simulink model "Wanderwellen_Leitungsmodell"  (R2022a)
settings: Solver=VariableStepAuto  StartTime=0.0  StopTime=0.05  RelTol=1e-3
model workspace (MAT data in the model file):
  C_impedanz = 1
  C_quelle = 1
  Delta_C = 2e-09
  Delta_G = 5000000
  Delta_L = 0.000228
  Delta_R = 0.048
  L_impedanz = 1
  L_quelle = 1
  R_impedanz = 0
  R_quelle = 0
  U = 20000
  U_type = 1
  Z_abschluss_type = 1
  Z_quelle_type = 1
  f = 50
  laenge = 0.2
  n_seg = 1
libraries: fl_lib x617, nesl_utility x207, ee_lib x3
(part 4 of 6)

== system Wanderwellen_Leitungsmodell/10 Leitungs-ESBs Nr. 3/Leitungs-ESB 6 ==
  Capacitor : fl_lib/Electrical/Electrical Elements/Capacitor  c=Delta_C F  r=1e-6 Ohm  g=0 1/Ohm  i_specify=off  i_priority=None  i=0 A  i_nominal_specify=off  i_nominal_unit=A  i_nominal_value=1  v_specify=off  v_priority=None  v=0 V  v_nominal_specify=off  v_nominal_unit=V  v_nominal_value=1  vc_specify=off  vc_priority=High  vc=0 V  vc_nominal_specify=off  vc_nominal_unit=V  vc_nominal_value=1
      settings: SourceProductBaseCode=PW,SS,VE
  Inductor : fl_lib/Electrical/Electrical Elements/Inductor  l=Delta_L H  r=0 Ohm  g=1e-9 1/Ohm  i_specify=off  i_priority=None  i=0 A  i_nominal_specify=off  i_nominal_unit=A  i_nominal_value=1  v_specify=off  v_priority=None  v=0 V  v_nominal_specify=off  v_nominal_unit=V  v_nominal_value=1  i_L_specify=off  i_L_priority=High  i_L=0 A  i_L_nominal_specify=off  i_L_nominal_unit=A  i_L_nominal_value=1
      settings: SourceProductBaseCode=PW,SS,VE
  Resistor : fl_lib/Electrical/Electrical Elements/Resistor  R=Delta_R Ohm  i_specify=off  i_priority=None  i=0 A  i_nominal_specify=off  i_nominal_unit=A  i_nominal_value=1  v_specify=off  v_priority=None  v=0 V  v_nominal_specify=off  v_nominal_unit=V  v_nominal_value=1
      settings: SourceProductBaseCode=PW,SS,VE
  Resistor1 : fl_lib/Electrical/Electrical Elements/Resistor  R=Delta_G Ohm  i_specify=off  i_priority=None  i=0 A  i_nominal_specify=off  i_nominal_unit=A  i_nominal_value=1  v_specify=off  v_priority=None  v=0 V  v_nominal_specify=off  v_nominal_unit=V  v_nominal_value=1
      settings: SourceProductBaseCode=PW,SS,VE
  L_in : PMIOPort  Side=Left
  N_in : PMIOPort  Port=2  Side=Left
  L_out : PMIOPort  Port=3  Side=Right
  N_out : PMIOPort  Port=4  Side=Right
  connections:
  Capacitor/LConn1 -- Resistor1/LConn1 -- Inductor/RConn1 -- L_out/RConn1
  Inductor/LConn1 -- Resistor/RConn1
  L_in/RConn1 -- Resistor/LConn1
  Resistor1/RConn1 -- N_in/RConn1 -- N_out/RConn1 -- Capacitor/RConn1

== system Wanderwellen_Leitungsmodell/10 Leitungs-ESBs Nr. 3/Leitungs-ESB 7 ==
  Capacitor : fl_lib/Electrical/Electrical Elements/Capacitor  c=Delta_C F  r=1e-6 Ohm  g=0 1/Ohm  i_specify=off  i_priority=None  i=0 A  i_nominal_specify=off  i_nominal_unit=A  i_nominal_value=1  v_specify=off  v_priority=None  v=0 V  v_nominal_specify=off  v_nominal_unit=V  v_nominal_value=1  vc_specify=off  vc_priority=High  vc=0 V  vc_nominal_specify=off  vc_nominal_unit=V  vc_nominal_value=1
      settings: SourceProductBaseCode=PW,SS,VE
  Inductor : fl_lib/Electrical/Electrical Elements/Inductor  l=Delta_L H  r=0 Ohm  g=1e-9 1/Ohm  i_specify=off  i_priority=None  i=0 A  i_nominal_specify=off  i_nominal_unit=A  i_nominal_value=1  v_specify=off  v_priority=None  v=0 V  v_nominal_specify=off  v_nominal_unit=V  v_nominal_value=1  i_L_specify=off  i_L_priority=High  i_L=0 A  i_L_nominal_specify=off  i_L_nominal_unit=A  i_L_nominal_value=1
      settings: SourceProductBaseCode=PW,SS,VE
  Resistor : fl_lib/Electrical/Electrical Elements/Resistor  R=Delta_R Ohm  i_specify=off  i_priority=None  i=0 A  i_nominal_specify=off  i_nominal_unit=A  i_nominal_value=1  v_specify=off  v_priority=None  v=0 V  v_nominal_specify=off  v_nominal_unit=V  v_nominal_value=1
      settings: SourceProductBaseCode=PW,SS,VE
  Resistor1 : fl_lib/Electrical/Electrical Elements/Resistor  R=Delta_G Ohm  i_specify=off  i_priority=None  i=0 A  i_nominal_specify=off  i_nominal_unit=A  i_nominal_value=1  v_specify=off  v_priority=None  v=0 V  v_nominal_specify=off  v_nominal_unit=V  v_nominal_value=1
      settings: SourceProductBaseCode=PW,SS,VE
  L_in : PMIOPort  Side=Left
  N_in : PMIOPort  Port=2  Side=Left
  L_out : PMIOPort  Port=3  Side=Right
  N_out : PMIOPort  Port=4  Side=Right
  connections:
  Capacitor/LConn1 -- Resistor1/LConn1 -- Inductor/RConn1 -- L_out/RConn1
  Inductor/LConn1 -- Resistor/RConn1
  L_in/RConn1 -- Resistor/LConn1
  Resistor1/RConn1 -- N_in/RConn1 -- N_out/RConn1 -- Capacitor/RConn1

== system Wanderwellen_Leitungsmodell/10 Leitungs-ESBs Nr. 3/Leitungs-ESB 8 ==
  Capacitor : fl_lib/Electrical/Electrical Elements/Capacitor  c=Delta_C F  r=1e-6 Ohm  g=0 1/Ohm  i_specify=off  i_priority=None  i=0 A  i_nominal_specify=off  i_nominal_unit=A  i_nominal_value=1  v_specify=off  v_priority=None  v=0 V  v_nominal_specify=off  v_nominal_unit=V  v_nominal_value=1  vc_specify=off  vc_priority=High  vc=0 V  vc_nominal_specify=off  vc_nominal_unit=V  vc_nominal_value=1
      settings: SourceProductBaseCode=PW,SS,VE
  Inductor : fl_lib/Electrical/Electrical Elements/Inductor  l=Delta_L H  r=0 Ohm  g=1e-9 1/Ohm  i_specify=off  i_priority=None  i=0 A  i_nominal_specify=off  i_nominal_unit=A  i_nominal_value=1  v_specify=off  v_priority=None  v=0 V  v_nominal_specify=off  v_nominal_unit=V  v_nominal_value=1  i_L_specify=off  i_L_priority=High  i_L=0 A  i_L_nominal_specify=off  i_L_nominal_unit=A  i_L_nominal_value=1
      settings: SourceProductBaseCode=PW,SS,VE
  Resistor : fl_lib/Electrical/Electrical Elements/Resistor  R=Delta_R Ohm  i_specify=off  i_priority=None  i=0 A  i_nominal_specify=off  i_nominal_unit=A  i_nominal_value=1  v_specify=off  v_priority=None  v=0 V  v_nominal_specify=off  v_nominal_unit=V  v_nominal_value=1
      settings: SourceProductBaseCode=PW,SS,VE
  Resistor1 : fl_lib/Electrical/Electrical Elements/Resistor  R=Delta_G Ohm  i_specify=off  i_priority=None  i=0 A  i_nominal_specify=off  i_nominal_unit=A  i_nominal_value=1  v_specify=off  v_priority=None  v=0 V  v_nominal_specify=off  v_nominal_unit=V  v_nominal_value=1
      settings: SourceProductBaseCode=PW,SS,VE
  L_in : PMIOPort  Side=Left
  N_in : PMIOPort  Port=2  Side=Left
  L_out : PMIOPort  Port=3  Side=Right
  N_out : PMIOPort  Port=4  Side=Right
  connections:
  Capacitor/LConn1 -- Resistor1/LConn1 -- Inductor/RConn1 -- L_out/RConn1
  Inductor/LConn1 -- Resistor/RConn1
  L_in/RConn1 -- Resistor/LConn1
  Resistor1/RConn1 -- N_in/RConn1 -- N_out/RConn1 -- Capacitor/RConn1

== system Wanderwellen_Leitungsmodell/10 Leitungs-ESBs Nr. 3/Leitungs-ESB 9 ==
  Capacitor : fl_lib/Electrical/Electrical Elements/Capacitor  c=Delta_C F  r=1e-6 Ohm  g=0 1/Ohm  i_specify=off  i_priority=None  i=0 A  i_nominal_specify=off  i_nominal_unit=A  i_nominal_value=1  v_specify=off  v_priority=None  v=0 V  v_nominal_specify=off  v_nominal_unit=V  v_nominal_value=1  vc_specify=off  vc_priority=High  vc=0 V  vc_nominal_specify=off  vc_nominal_unit=V  vc_nominal_value=1
      settings: SourceProductBaseCode=PW,SS,VE
  Inductor : fl_lib/Electrical/Electrical Elements/Inductor  l=Delta_L H  r=0 Ohm  g=1e-9 1/Ohm  i_specify=off  i_priority=None  i=0 A  i_nominal_specify=off  i_nominal_unit=A  i_nominal_value=1  v_specify=off  v_priority=None  v=0 V  v_nominal_specify=off  v_nominal_unit=V  v_nominal_value=1  i_L_specify=off  i_L_priority=High  i_L=0 A  i_L_nominal_specify=off  i_L_nominal_unit=A  i_L_nominal_value=1
      settings: SourceProductBaseCode=PW,SS,VE
  Resistor : fl_lib/Electrical/Electrical Elements/Resistor  R=Delta_R Ohm  i_specify=off  i_priority=None  i=0 A  i_nominal_specify=off  i_nominal_unit=A  i_nominal_value=1  v_specify=off  v_priority=None  v=0 V  v_nominal_specify=off  v_nominal_unit=V  v_nominal_value=1
      settings: SourceProductBaseCode=PW,SS,VE
  Resistor1 : fl_lib/Electrical/Electrical Elements/Resistor  R=Delta_G Ohm  i_specify=off  i_priority=None  i=0 A  i_nominal_specify=off  i_nominal_unit=A  i_nominal_value=1  v_specify=off  v_priority=None  v=0 V  v_nominal_specify=off  v_nominal_unit=V  v_nominal_value=1
      settings: SourceProductBaseCode=PW,SS,VE
  L_in : PMIOPort  Side=Left
  N_in : PMIOPort  Port=2  Side=Left
  L_out : PMIOPort  Port=3  Side=Right
  N_out : PMIOPort  Port=4  Side=Right
  connections:
  Capacitor/LConn1 -- Resistor1/LConn1 -- Inductor/RConn1 -- L_out/RConn1
  Inductor/LConn1 -- Resistor/RConn1
  L_in/RConn1 -- Resistor/LConn1
  Resistor1/RConn1 -- N_in/RConn1 -- N_out/RConn1 -- Capacitor/RConn1

== system Wanderwellen_Leitungsmodell/10 Leitungs-ESBs Nr. 4/Leitungs-ESB 1 ==
  Capacitor : fl_lib/Electrical/Electrical Elements/Capacitor  c=Delta_C F  r=1e-6 Ohm  g=0 1/Ohm  i_specify=off  i_priority=None  i=0 A  i_nominal_specify=off  i_nominal_unit=A  i_nominal_value=1  v_specify=off  v_priority=None  v=0 V  v_nominal_specify=off  v_nominal_unit=V  v_nominal_value=1  vc_specify=off  vc_priority=High  vc=0 V  vc_nominal_specify=off  vc_nominal_unit=V  vc_nominal_value=1
      settings: SourceProductBaseCode=PW,SS,VE
  Inductor : fl_lib/Electrical/Electrical Elements/Inductor  l=Delta_L H  r=0 Ohm  g=1e-9 1/Ohm  i_specify=off  i_priority=None  i=0 A  i_nominal_specify=off  i_nominal_unit=A  i_nominal_value=1  v_specify=off  v_priority=None  v=0 V  v_nominal_specify=off  v_nominal_unit=V  v_nominal_value=1  i_L_specify=off  i_L_priority=High  i_L=0 A  i_L_nominal_specify=off  i_L_nominal_unit=A  i_L_nominal_value=1
      settings: SourceProductBaseCode=PW,SS,VE
  Resistor : fl_lib/Electrical/Electrical Elements/Resistor  R=Delta_R Ohm  i_specify=off  i_priority=None  i=0 A  i_nominal_specify=off  i_nominal_unit=A  i_nominal_value=1  v_specify=off  v_priority=None  v=0 V  v_nominal_specify=off  v_nominal_unit=V  v_nominal_value=1
      settings: SourceProductBaseCode=PW,SS,VE
  Resistor1 : fl_lib/Electrical/Electrical Elements/Resistor  R=Delta_G Ohm  i_specify=off  i_priority=None  i=0 A  i_nominal_specify=off  i_nominal_unit=A  i_nominal_value=1  v_specify=off  v_priority=None  v=0 V  v_nominal_specify=off  v_nominal_unit=V  v_nominal_value=1
      settings: SourceProductBaseCode=PW,SS,VE
  L_in : PMIOPort  Side=Left
  N_in : PMIOPort  Port=2  Side=Left
  L_out : PMIOPort  Port=3  Side=Right
  N_out : PMIOPort  Port=4  Side=Right
  connections:
  Capacitor/LConn1 -- Resistor1/LConn1 -- Inductor/RConn1 -- L_out/RConn1
  Inductor/LConn1 -- Resistor/RConn1
  L_in/RConn1 -- Resistor/LConn1
  Resistor1/RConn1 -- N_in/RConn1 -- N_out/RConn1 -- Capacitor/RConn1

== system Wanderwellen_Leitungsmodell/10 Leitungs-ESBs Nr. 4/Leitungs-ESB 10 ==
  Capacitor : fl_lib/Electrical/Electrical Elements/Capacitor  c=Delta_C F  r=1e-6 Ohm  g=0 1/Ohm  i_specify=off  i_priority=None  i=0 A  i_nominal_specify=off  i_nominal_unit=A  i_nominal_value=1  v_specify=off  v_priority=None  v=0 V  v_nominal_specify=off  v_nominal_unit=V  v_nominal_value=1  vc_specify=off  vc_priority=High  vc=0 V  vc_nominal_specify=off  vc_nominal_unit=V  vc_nominal_value=1
      settings: SourceProductBaseCode=PW,SS,VE
  Inductor : fl_lib/Electrical/Electrical Elements/Inductor  l=Delta_L H  r=0 Ohm  g=1e-9 1/Ohm  i_specify=off  i_priority=None  i=0 A  i_nominal_specify=off  i_nominal_unit=A  i_nominal_value=1  v_specify=off  v_priority=None  v=0 V  v_nominal_specify=off  v_nominal_unit=V  v_nominal_value=1  i_L_specify=off  i_L_priority=High  i_L=0 A  i_L_nominal_specify=off  i_L_nominal_unit=A  i_L_nominal_value=1
      settings: SourceProductBaseCode=PW,SS,VE
  Resistor : fl_lib/Electrical/Electrical Elements/Resistor  R=Delta_R Ohm  i_specify=off  i_priority=None  i=0 A  i_nominal_specify=off  i_nominal_unit=A  i_nominal_value=1  v_specify=off  v_priority=None  v=0 V  v_nominal_specify=off  v_nominal_unit=V  v_nominal_value=1
      settings: SourceProductBaseCode=PW,SS,VE
  Resistor1 : fl_lib/Electrical/Electrical Elements/Resistor  R=Delta_G Ohm  i_specify=off  i_priority=None  i=0 A  i_nominal_specify=off  i_nominal_unit=A  i_nominal_value=1  v_specify=off  v_priority=None  v=0 V  v_nominal_specify=off  v_nominal_unit=V  v_nominal_value=1
      settings: SourceProductBaseCode=PW,SS,VE
  L_in : PMIOPort  Side=Left
  N_in : PMIOPort  Port=2  Side=Left
  L_out : PMIOPort  Port=3  Side=Right
  N_out : PMIOPort  Port=4  Side=Right
  connections:
  Capacitor/LConn1 -- Resistor1/LConn1 -- Inductor/RConn1 -- L_out/RConn1
  Inductor/LConn1 -- Resistor/RConn1
  L_in/RConn1 -- Resistor/LConn1
  Resistor1/RConn1 -- N_in/RConn1 -- N_out/RConn1 -- Capacitor/RConn1

== system Wanderwellen_Leitungsmodell/10 Leitungs-ESBs Nr. 4/Leitungs-ESB 2 ==
  Capacitor : fl_lib/Electrical/Electrical Elements/Capacitor  c=Delta_C F  r=1e-6 Ohm  g=0 1/Ohm  i_specify=off  i_priority=None  i=0 A  i_nominal_specify=off  i_nominal_unit=A  i_nominal_value=1  v_specify=off  v_priority=None  v=0 V  v_nominal_specify=off  v_nominal_unit=V  v_nominal_value=1  vc_specify=off  vc_priority=High  vc=0 V  vc_nominal_specify=off  vc_nominal_unit=V  vc_nominal_value=1
      settings: SourceProductBaseCode=PW,SS,VE
  Inductor : fl_lib/Electrical/Electrical Elements/Inductor  l=Delta_L H  r=0 Ohm  g=1e-9 1/Ohm  i_specify=off  i_priority=None  i=0 A  i_nominal_specify=off  i_nominal_unit=A  i_nominal_value=1  v_specify=off  v_priority=None  v=0 V  v_nominal_specify=off  v_nominal_unit=V  v_nominal_value=1  i_L_specify=off  i_L_priority=High  i_L=0 A  i_L_nominal_specify=off  i_L_nominal_unit=A  i_L_nominal_value=1
      settings: SourceProductBaseCode=PW,SS,VE
  Resistor : fl_lib/Electrical/Electrical Elements/Resistor  R=Delta_R Ohm  i_specify=off  i_priority=None  i=0 A  i_nominal_specify=off  i_nominal_unit=A  i_nominal_value=1  v_specify=off  v_priority=None  v=0 V  v_nominal_specify=off  v_nominal_unit=V  v_nominal_value=1
      settings: SourceProductBaseCode=PW,SS,VE
  Resistor1 : fl_lib/Electrical/Electrical Elements/Resistor  R=Delta_G Ohm  i_specify=off  i_priority=None  i=0 A  i_nominal_specify=off  i_nominal_unit=A  i_nominal_value=1  v_specify=off  v_priority=None  v=0 V  v_nominal_specify=off  v_nominal_unit=V  v_nominal_value=1
      settings: SourceProductBaseCode=PW,SS,VE
  L_in : PMIOPort  Side=Left
  N_in : PMIOPort  Port=2  Side=Left
  L_out : PMIOPort  Port=3  Side=Right
  N_out : PMIOPort  Port=4  Side=Right
  connections:
  Capacitor/LConn1 -- Resistor1/LConn1 -- Inductor/RConn1 -- L_out/RConn1
  Inductor/LConn1 -- Resistor/RConn1
  L_in/RConn1 -- Resistor/LConn1
  Resistor1/RConn1 -- N_in/RConn1 -- N_out/RConn1 -- Capacitor/RConn1

== system Wanderwellen_Leitungsmodell/10 Leitungs-ESBs Nr. 4/Leitungs-ESB 3 ==
  Capacitor : fl_lib/Electrical/Electrical Elements/Capacitor  c=Delta_C F  r=1e-6 Ohm  g=0 1/Ohm  i_specify=off  i_priority=None  i=0 A  i_nominal_specify=off  i_nominal_unit=A  i_nominal_value=1  v_specify=off  v_priority=None  v=0 V  v_nominal_specify=off  v_nominal_unit=V  v_nominal_value=1  vc_specify=off  vc_priority=High  vc=0 V  vc_nominal_specify=off  vc_nominal_unit=V  vc_nominal_value=1
      settings: SourceProductBaseCode=PW,SS,VE
  Inductor : fl_lib/Electrical/Electrical Elements/Inductor  l=Delta_L H  r=0 Ohm  g=1e-9 1/Ohm  i_specify=off  i_priority=None  i=0 A  i_nominal_specify=off  i_nominal_unit=A  i_nominal_value=1  v_specify=off  v_priority=None  v=0 V  v_nominal_specify=off  v_nominal_unit=V  v_nominal_value=1  i_L_specify=off  i_L_priority=High  i_L=0 A  i_L_nominal_specify=off  i_L_nominal_unit=A  i_L_nominal_value=1
      settings: SourceProductBaseCode=PW,SS,VE
  Resistor : fl_lib/Electrical/Electrical Elements/Resistor  R=Delta_R Ohm  i_specify=off  i_priority=None  i=0 A  i_nominal_specify=off  i_nominal_unit=A  i_nominal_value=1  v_specify=off  v_priority=None  v=0 V  v_nominal_specify=off  v_nominal_unit=V  v_nominal_value=1
      settings: SourceProductBaseCode=PW,SS,VE
  Resistor1 : fl_lib/Electrical/Electrical Elements/Resistor  R=Delta_G Ohm  i_specify=off  i_priority=None  i=0 A  i_nominal_specify=off  i_nominal_unit=A  i_nominal_value=1  v_specify=off  v_priority=None  v=0 V  v_nominal_specify=off  v_nominal_unit=V  v_nominal_value=1
      settings: SourceProductBaseCode=PW,SS,VE
  L_in : PMIOPort  Side=Left
  N_in : PMIOPort  Port=2  Side=Left
  L_out : PMIOPort  Port=3  Side=Right
  N_out : PMIOPort  Port=4  Side=Right
  connections:
  Capacitor/LConn1 -- Resistor1/LConn1 -- Inductor/RConn1 -- L_out/RConn1
  Inductor/LConn1 -- Resistor/RConn1
  L_in/RConn1 -- Resistor/LConn1
  Resistor1/RConn1 -- N_in/RConn1 -- N_out/RConn1 -- Capacitor/RConn1

== system Wanderwellen_Leitungsmodell/10 Leitungs-ESBs Nr. 4/Leitungs-ESB 4 ==
  Capacitor : fl_lib/Electrical/Electrical Elements/Capacitor  c=Delta_C F  r=1e-6 Ohm  g=0 1/Ohm  i_specify=off  i_priority=None  i=0 A  i_nominal_specify=off  i_nominal_unit=A  i_nominal_value=1  v_specify=off  v_priority=None  v=0 V  v_nominal_specify=off  v_nominal_unit=V  v_nominal_value=1  vc_specify=off  vc_priority=High  vc=0 V  vc_nominal_specify=off  vc_nominal_unit=V  vc_nominal_value=1
      settings: SourceProductBaseCode=PW,SS,VE
  Inductor : fl_lib/Electrical/Electrical Elements/Inductor  l=Delta_L H  r=0 Ohm  g=1e-9 1/Ohm  i_specify=off  i_priority=None  i=0 A  i_nominal_specify=off  i_nominal_unit=A  i_nominal_value=1  v_specify=off  v_priority=None  v=0 V  v_nominal_specify=off  v_nominal_unit=V  v_nominal_value=1  i_L_specify=off  i_L_priority=High  i_L=0 A  i_L_nominal_specify=off  i_L_nominal_unit=A  i_L_nominal_value=1
      settings: SourceProductBaseCode=PW,SS,VE
  Resistor : fl_lib/Electrical/Electrical Elements/Resistor  R=Delta_R Ohm  i_specify=off  i_priority=None  i=0 A  i_nominal_specify=off  i_nominal_unit=A  i_nominal_value=1  v_specify=off  v_priority=None  v=0 V  v_nominal_specify=off  v_nominal_unit=V  v_nominal_value=1
      settings: SourceProductBaseCode=PW,SS,VE
  Resistor1 : fl_lib/Electrical/Electrical Elements/Resistor  R=Delta_G Ohm  i_specify=off  i_priority=None  i=0 A  i_nominal_specify=off  i_nominal_unit=A  i_nominal_value=1  v_specify=off  v_priority=None  v=0 V  v_nominal_specify=off  v_nominal_unit=V  v_nominal_value=1
      settings: SourceProductBaseCode=PW,SS,VE
  L_in : PMIOPort  Side=Left
  N_in : PMIOPort  Port=2  Side=Left
  L_out : PMIOPort  Port=3  Side=Right
  N_out : PMIOPort  Port=4  Side=Right
  connections:
  Capacitor/LConn1 -- Resistor1/LConn1 -- Inductor/RConn1 -- L_out/RConn1
  Inductor/LConn1 -- Resistor/RConn1
  L_in/RConn1 -- Resistor/LConn1
  Resistor1/RConn1 -- N_in/RConn1 -- N_out/RConn1 -- Capacitor/RConn1

== system Wanderwellen_Leitungsmodell/10 Leitungs-ESBs Nr. 4/Leitungs-ESB 5 ==
  Capacitor : fl_lib/Electrical/Electrical Elements/Capacitor  c=Delta_C F  r=1e-6 Ohm  g=0 1/Ohm  i_specify=off  i_priority=None  i=0 A  i_nominal_specify=off  i_nominal_unit=A  i_nominal_value=1  v_specify=off  v_priority=None  v=0 V  v_nominal_specify=off  v_nominal_unit=V  v_nominal_value=1  vc_specify=off  vc_priority=High  vc=0 V  vc_nominal_specify=off  vc_nominal_unit=V  vc_nominal_value=1
      settings: SourceProductBaseCode=PW,SS,VE
  Inductor : fl_lib/Electrical/Electrical Elements/Inductor  l=Delta_L H  r=0 Ohm  g=1e-9 1/Ohm  i_specify=off  i_priority=None  i=0 A  i_nominal_specify=off  i_nominal_unit=A  i_nominal_value=1  v_specify=off  v_priority=None  v=0 V  v_nominal_specify=off  v_nominal_unit=V  v_nominal_value=1  i_L_specify=off  i_L_priority=High  i_L=0 A  i_L_nominal_specify=off  i_L_nominal_unit=A  i_L_nominal_value=1
      settings: SourceProductBaseCode=PW,SS,VE
  Resistor : fl_lib/Electrical/Electrical Elements/Resistor  R=Delta_R Ohm  i_specify=off  i_priority=None  i=0 A  i_nominal_specify=off  i_nominal_unit=A  i_nominal_value=1  v_specify=off  v_priority=None  v=0 V  v_nominal_specify=off  v_nominal_unit=V  v_nominal_value=1
      settings: SourceProductBaseCode=PW,SS,VE
  Resistor1 : fl_lib/Electrical/Electrical Elements/Resistor  R=Delta_G Ohm  i_specify=off  i_priority=None  i=0 A  i_nominal_specify=off  i_nominal_unit=A  i_nominal_value=1  v_specify=off  v_priority=None  v=0 V  v_nominal_specify=off  v_nominal_unit=V  v_nominal_value=1
      settings: SourceProductBaseCode=PW,SS,VE
  L_in : PMIOPort  Side=Left
  N_in : PMIOPort  Port=2  Side=Left
  L_out : PMIOPort  Port=3  Side=Right
  N_out : PMIOPort  Port=4  Side=Right
  connections:
  Capacitor/LConn1 -- Resistor1/LConn1 -- Inductor/RConn1 -- L_out/RConn1
  Inductor/LConn1 -- Resistor/RConn1
  L_in/RConn1 -- Resistor/LConn1
  Resistor1/RConn1 -- N_in/RConn1 -- N_out/RConn1 -- Capacitor/RConn1

== system Wanderwellen_Leitungsmodell/10 Leitungs-ESBs Nr. 4/Leitungs-ESB 6 ==
  Capacitor : fl_lib/Electrical/Electrical Elements/Capacitor  c=Delta_C F  r=1e-6 Ohm  g=0 1/Ohm  i_specify=off  i_priority=None  i=0 A  i_nominal_specify=off  i_nominal_unit=A  i_nominal_value=1  v_specify=off  v_priority=None  v=0 V  v_nominal_specify=off  v_nominal_unit=V  v_nominal_value=1  vc_specify=off  vc_priority=High  vc=0 V  vc_nominal_specify=off  vc_nominal_unit=V  vc_nominal_value=1
      settings: SourceProductBaseCode=PW,SS,VE
  Inductor : fl_lib/Electrical/Electrical Elements/Inductor  l=Delta_L H  r=0 Ohm  g=1e-9 1/Ohm  i_specify=off  i_priority=None  i=0 A  i_nominal_specify=off  i_nominal_unit=A  i_nominal_value=1  v_specify=off  v_priority=None  v=0 V  v_nominal_specify=off  v_nominal_unit=V  v_nominal_value=1  i_L_specify=off  i_L_priority=High  i_L=0 A  i_L_nominal_specify=off  i_L_nominal_unit=A  i_L_nominal_value=1
      settings: SourceProductBaseCode=PW,SS,VE
  Resistor : fl_lib/Electrical/Electrical Elements/Resistor  R=Delta_R Ohm  i_specify=off  i_priority=None  i=0 A  i_nominal_specify=off  i_nominal_unit=A  i_nominal_value=1  v_specify=off  v_priority=None  v=0 V  v_nominal_specify=off  v_nominal_unit=V  v_nominal_value=1
      settings: SourceProductBaseCode=PW,SS,VE
  Resistor1 : fl_lib/Electrical/Electrical Elements/Resistor  R=Delta_G Ohm  i_specify=off  i_priority=None  i=0 A  i_nominal_specify=off  i_nominal_unit=A  i_nominal_value=1  v_specify=off  v_priority=None  v=0 V  v_nominal_specify=off  v_nominal_unit=V  v_nominal_value=1
      settings: SourceProductBaseCode=PW,SS,VE
  L_in : PMIOPort  Side=Left
  N_in : PMIOPort  Port=2  Side=Left
  L_out : PMIOPort  Port=3  Side=Right
  N_out : PMIOPort  Port=4  Side=Right
  connections:
  Capacitor/LConn1 -- Resistor1/LConn1 -- Inductor/RConn1 -- L_out/RConn1
  Inductor/LConn1 -- Resistor/RConn1
  L_in/RConn1 -- Resistor/LConn1
  Resistor1/RConn1 -- N_in/RConn1 -- N_out/RConn1 -- Capacitor/RConn1

== system Wanderwellen_Leitungsmodell/10 Leitungs-ESBs Nr. 4/Leitungs-ESB 7 ==
  Capacitor : fl_lib/Electrical/Electrical Elements/Capacitor  c=Delta_C F  r=1e-6 Ohm  g=0 1/Ohm  i_specify=off  i_priority=None  i=0 A  i_nominal_specify=off  i_nominal_unit=A  i_nominal_value=1  v_specify=off  v_priority=None  v=0 V  v_nominal_specify=off  v_nominal_unit=V  v_nominal_value=1  vc_specify=off  vc_priority=High  vc=0 V  vc_nominal_specify=off  vc_nominal_unit=V  vc_nominal_value=1
      settings: SourceProductBaseCode=PW,SS,VE
  Inductor : fl_lib/Electrical/Electrical Elements/Inductor  l=Delta_L H  r=0 Ohm  g=1e-9 1/Ohm  i_specify=off  i_priority=None  i=0 A  i_nominal_specify=off  i_nominal_unit=A  i_nominal_value=1  v_specify=off  v_priority=None  v=0 V  v_nominal_specify=off  v_nominal_unit=V  v_nominal_value=1  i_L_specify=off  i_L_priority=High  i_L=0 A  i_L_nominal_specify=off  i_L_nominal_unit=A  i_L_nominal_value=1
      settings: SourceProductBaseCode=PW,SS,VE
  Resistor : fl_lib/Electrical/Electrical Elements/Resistor  R=Delta_R Ohm  i_specify=off  i_priority=None  i=0 A  i_nominal_specify=off  i_nominal_unit=A  i_nominal_value=1  v_specify=off  v_priority=None  v=0 V  v_nominal_specify=off  v_nominal_unit=V  v_nominal_value=1
      settings: SourceProductBaseCode=PW,SS,VE
  Resistor1 : fl_lib/Electrical/Electrical Elements/Resistor  R=Delta_G Ohm  i_specify=off  i_priority=None  i=0 A  i_nominal_specify=off  i_nominal_unit=A  i_nominal_value=1  v_specify=off  v_priority=None  v=0 V  v_nominal_specify=off  v_nominal_unit=V  v_nominal_value=1
      settings: SourceProductBaseCode=PW,SS,VE
  L_in : PMIOPort  Side=Left
  N_in : PMIOPort  Port=2  Side=Left
  L_out : PMIOPort  Port=3  Side=Right
  N_out : PMIOPort  Port=4  Side=Right
  connections:
  Capacitor/LConn1 -- Resistor1/LConn1 -- Inductor/RConn1 -- L_out/RConn1
  Inductor/LConn1 -- Resistor/RConn1
  L_in/RConn1 -- Resistor/LConn1
  Resistor1/RConn1 -- N_in/RConn1 -- N_out/RConn1 -- Capacitor/RConn1

== system Wanderwellen_Leitungsmodell/10 Leitungs-ESBs Nr. 4/Leitungs-ESB 8 ==
  Capacitor : fl_lib/Electrical/Electrical Elements/Capacitor  c=Delta_C F  r=1e-6 Ohm  g=0 1/Ohm  i_specify=off  i_priority=None  i=0 A  i_nominal_specify=off  i_nominal_unit=A  i_nominal_value=1  v_specify=off  v_priority=None  v=0 V  v_nominal_specify=off  v_nominal_unit=V  v_nominal_value=1  vc_specify=off  vc_priority=High  vc=0 V  vc_nominal_specify=off  vc_nominal_unit=V  vc_nominal_value=1
      settings: SourceProductBaseCode=PW,SS,VE
  Inductor : fl_lib/Electrical/Electrical Elements/Inductor  l=Delta_L H  r=0 Ohm  g=1e-9 1/Ohm  i_specify=off  i_priority=None  i=0 A  i_nominal_specify=off  i_nominal_unit=A  i_nominal_value=1  v_specify=off  v_priority=None  v=0 V  v_nominal_specify=off  v_nominal_unit=V  v_nominal_value=1  i_L_specify=off  i_L_priority=High  i_L=0 A  i_L_nominal_specify=off  i_L_nominal_unit=A  i_L_nominal_value=1
      settings: SourceProductBaseCode=PW,SS,VE
  Resistor : fl_lib/Electrical/Electrical Elements/Resistor  R=Delta_R Ohm  i_specify=off  i_priority=None  i=0 A  i_nominal_specify=off  i_nominal_unit=A  i_nominal_value=1  v_specify=off  v_priority=None  v=0 V  v_nominal_specify=off  v_nominal_unit=V  v_nominal_value=1
      settings: SourceProductBaseCode=PW,SS,VE
  Resistor1 : fl_lib/Electrical/Electrical Elements/Resistor  R=Delta_G Ohm  i_specify=off  i_priority=None  i=0 A  i_nominal_specify=off  i_nominal_unit=A  i_nominal_value=1  v_specify=off  v_priority=None  v=0 V  v_nominal_specify=off  v_nominal_unit=V  v_nominal_value=1
      settings: SourceProductBaseCode=PW,SS,VE
  L_in : PMIOPort  Side=Left
  N_in : PMIOPort  Port=2  Side=Left
  L_out : PMIOPort  Port=3  Side=Right
  N_out : PMIOPort  Port=4  Side=Right
  connections:
  Capacitor/LConn1 -- Resistor1/LConn1 -- Inductor/RConn1 -- L_out/RConn1
  Inductor/LConn1 -- Resistor/RConn1
  L_in/RConn1 -- Resistor/LConn1
  Resistor1/RConn1 -- N_in/RConn1 -- N_out/RConn1 -- Capacitor/RConn1

== system Wanderwellen_Leitungsmodell/10 Leitungs-ESBs Nr. 4/Leitungs-ESB 9 ==
  Capacitor : fl_lib/Electrical/Electrical Elements/Capacitor  c=Delta_C F  r=1e-6 Ohm  g=0 1/Ohm  i_specify=off  i_priority=None  i=0 A  i_nominal_specify=off  i_nominal_unit=A  i_nominal_value=1  v_specify=off  v_priority=None  v=0 V  v_nominal_specify=off  v_nominal_unit=V  v_nominal_value=1  vc_specify=off  vc_priority=High  vc=0 V  vc_nominal_specify=off  vc_nominal_unit=V  vc_nominal_value=1
      settings: SourceProductBaseCode=PW,SS,VE
  Inductor : fl_lib/Electrical/Electrical Elements/Inductor  l=Delta_L H  r=0 Ohm  g=1e-9 1/Ohm  i_specify=off  i_priority=None  i=0 A  i_nominal_specify=off  i_nominal_unit=A  i_nominal_value=1  v_specify=off  v_priority=None  v=0 V  v_nominal_specify=off  v_nominal_unit=V  v_nominal_value=1  i_L_specify=off  i_L_priority=High  i_L=0 A  i_L_nominal_specify=off  i_L_nominal_unit=A  i_L_nominal_value=1
      settings: SourceProductBaseCode=PW,SS,VE
  Resistor : fl_lib/Electrical/Electrical Elements/Resistor  R=Delta_R Ohm  i_specify=off  i_priority=None  i=0 A  i_nominal_specify=off  i_nominal_unit=A  i_nominal_value=1  v_specify=off  v_priority=None  v=0 V  v_nominal_specify=off  v_nominal_unit=V  v_nominal_value=1
      settings: SourceProductBaseCode=PW,SS,VE
  Resistor1 : fl_lib/Electrical/Electrical Elements/Resistor  R=Delta_G Ohm  i_specify=off  i_priority=None  i=0 A  i_nominal_specify=off  i_nominal_unit=A  i_nominal_value=1  v_specify=off  v_priority=None  v=0 V  v_nominal_specify=off  v_nominal_unit=V  v_nominal_value=1
      settings: SourceProductBaseCode=PW,SS,VE
  L_in : PMIOPort  Side=Left
  N_in : PMIOPort  Port=2  Side=Left
  L_out : PMIOPort  Port=3  Side=Right
  N_out : PMIOPort  Port=4  Side=Right
  connections:
  Capacitor/LConn1 -- Resistor1/LConn1 -- Inductor/RConn1 -- L_out/RConn1
  Inductor/LConn1 -- Resistor/RConn1
  L_in/RConn1 -- Resistor/LConn1
  Resistor1/RConn1 -- N_in/RConn1 -- N_out/RConn1 -- Capacitor/RConn1

== system Wanderwellen_Leitungsmodell/10 Leitungs-ESBs Nr. 5/Leitungs-ESB 1 ==
  Capacitor : fl_lib/Electrical/Electrical Elements/Capacitor  c=Delta_C F  r=1e-6 Ohm  g=0 1/Ohm  i_specify=off  i_priority=None  i=0 A  i_nominal_specify=off  i_nominal_unit=A  i_nominal_value=1  v_specify=off  v_priority=None  v=0 V  v_nominal_specify=off  v_nominal_unit=V  v_nominal_value=1  vc_specify=off  vc_priority=High  vc=0 V  vc_nominal_specify=off  vc_nominal_unit=V  vc_nominal_value=1
      settings: SourceProductBaseCode=PW,SS,VE
  Inductor : fl_lib/Electrical/Electrical Elements/Inductor  l=Delta_L H  r=0 Ohm  g=1e-9 1/Ohm  i_specify=off  i_priority=None  i=0 A  i_nominal_specify=off  i_nominal_unit=A  i_nominal_value=1  v_specify=off  v_priority=None  v=0 V  v_nominal_specify=off  v_nominal_unit=V  v_nominal_value=1  i_L_specify=off  i_L_priority=High  i_L=0 A  i_L_nominal_specify=off  i_L_nominal_unit=A  i_L_nominal_value=1
      settings: SourceProductBaseCode=PW,SS,VE
  Resistor : fl_lib/Electrical/Electrical Elements/Resistor  R=Delta_R Ohm  i_specify=off  i_priority=None  i=0 A  i_nominal_specify=off  i_nominal_unit=A  i_nominal_value=1  v_specify=off  v_priority=None  v=0 V  v_nominal_specify=off  v_nominal_unit=V  v_nominal_value=1
      settings: SourceProductBaseCode=PW,SS,VE
  Resistor1 : fl_lib/Electrical/Electrical Elements/Resistor  R=Delta_G Ohm  i_specify=off  i_priority=None  i=0 A  i_nominal_specify=off  i_nominal_unit=A  i_nominal_value=1  v_specify=off  v_priority=None  v=0 V  v_nominal_specify=off  v_nominal_unit=V  v_nominal_value=1
      settings: SourceProductBaseCode=PW,SS,VE
  L_in : PMIOPort  Side=Left
  N_in : PMIOPort  Port=2  Side=Left
  L_out : PMIOPort  Port=3  Side=Right
  N_out : PMIOPort  Port=4  Side=Right
  connections:
  Capacitor/LConn1 -- Resistor1/LConn1 -- Inductor/RConn1 -- L_out/RConn1
  Inductor/LConn1 -- Resistor/RConn1
  L_in/RConn1 -- Resistor/LConn1
  Resistor1/RConn1 -- N_in/RConn1 -- N_out/RConn1 -- Capacitor/RConn1

== system Wanderwellen_Leitungsmodell/10 Leitungs-ESBs Nr. 5/Leitungs-ESB 10 ==
  Capacitor : fl_lib/Electrical/Electrical Elements/Capacitor  c=Delta_C F  r=1e-6 Ohm  g=0 1/Ohm  i_specify=off  i_priority=None  i=0 A  i_nominal_specify=off  i_nominal_unit=A  i_nominal_value=1  v_specify=off  v_priority=None  v=0 V  v_nominal_specify=off  v_nominal_unit=V  v_nominal_value=1  vc_specify=off  vc_priority=High  vc=0 V  vc_nominal_specify=off  vc_nominal_unit=V  vc_nominal_value=1
      settings: SourceProductBaseCode=PW,SS,VE
  Inductor : fl_lib/Electrical/Electrical Elements/Inductor  l=Delta_L H  r=0 Ohm  g=1e-9 1/Ohm  i_specify=off  i_priority=None  i=0 A  i_nominal_specify=off  i_nominal_unit=A  i_nominal_value=1  v_specify=off  v_priority=None  v=0 V  v_nominal_specify=off  v_nominal_unit=V  v_nominal_value=1  i_L_specify=off  i_L_priority=High  i_L=0 A  i_L_nominal_specify=off  i_L_nominal_unit=A  i_L_nominal_value=1
      settings: SourceProductBaseCode=PW,SS,VE
  Resistor : fl_lib/Electrical/Electrical Elements/Resistor  R=Delta_R Ohm  i_specify=off  i_priority=None  i=0 A  i_nominal_specify=off  i_nominal_unit=A  i_nominal_value=1  v_specify=off  v_priority=None  v=0 V  v_nominal_specify=off  v_nominal_unit=V  v_nominal_value=1
      settings: SourceProductBaseCode=PW,SS,VE
  Resistor1 : fl_lib/Electrical/Electrical Elements/Resistor  R=Delta_G Ohm  i_specify=off  i_priority=None  i=0 A  i_nominal_specify=off  i_nominal_unit=A  i_nominal_value=1  v_specify=off  v_priority=None  v=0 V  v_nominal_specify=off  v_nominal_unit=V  v_nominal_value=1
      settings: SourceProductBaseCode=PW,SS,VE
  L_in : PMIOPort  Side=Left
  N_in : PMIOPort  Port=2  Side=Left
  L_out : PMIOPort  Port=3  Side=Right
  N_out : PMIOPort  Port=4  Side=Right
  connections:
  Capacitor/LConn1 -- Resistor1/LConn1 -- Inductor/RConn1 -- L_out/RConn1
  Inductor/LConn1 -- Resistor/RConn1
  L_in/RConn1 -- Resistor/LConn1
  Resistor1/RConn1 -- N_in/RConn1 -- N_out/RConn1 -- Capacitor/RConn1

== system Wanderwellen_Leitungsmodell/10 Leitungs-ESBs Nr. 5/Leitungs-ESB 2 ==
  Capacitor : fl_lib/Electrical/Electrical Elements/Capacitor  c=Delta_C F  r=1e-6 Ohm  g=0 1/Ohm  i_specify=off  i_priority=None  i=0 A  i_nominal_specify=off  i_nominal_unit=A  i_nominal_value=1  v_specify=off  v_priority=None  v=0 V  v_nominal_specify=off  v_nominal_unit=V  v_nominal_value=1  vc_specify=off  vc_priority=High  vc=0 V  vc_nominal_specify=off  vc_nominal_unit=V  vc_nominal_value=1
      settings: SourceProductBaseCode=PW,SS,VE
  Inductor : fl_lib/Electrical/Electrical Elements/Inductor  l=Delta_L H  r=0 Ohm  g=1e-9 1/Ohm  i_specify=off  i_priority=None  i=0 A  i_nominal_specify=off  i_nominal_unit=A  i_nominal_value=1  v_specify=off  v_priority=None  v=0 V  v_nominal_specify=off  v_nominal_unit=V  v_nominal_value=1  i_L_specify=off  i_L_priority=High  i_L=0 A  i_L_nominal_specify=off  i_L_nominal_unit=A  i_L_nominal_value=1
      settings: SourceProductBaseCode=PW,SS,VE
  Resistor : fl_lib/Electrical/Electrical Elements/Resistor  R=Delta_R Ohm  i_specify=off  i_priority=None  i=0 A  i_nominal_specify=off  i_nominal_unit=A  i_nominal_value=1  v_specify=off  v_priority=None  v=0 V  v_nominal_specify=off  v_nominal_unit=V  v_nominal_value=1
      settings: SourceProductBaseCode=PW,SS,VE
  Resistor1 : fl_lib/Electrical/Electrical Elements/Resistor  R=Delta_G Ohm  i_specify=off  i_priority=None  i=0 A  i_nominal_specify=off  i_nominal_unit=A  i_nominal_value=1  v_specify=off  v_priority=None  v=0 V  v_nominal_specify=off  v_nominal_unit=V  v_nominal_value=1
      settings: SourceProductBaseCode=PW,SS,VE
  L_in : PMIOPort  Side=Left
  N_in : PMIOPort  Port=2  Side=Left
  L_out : PMIOPort  Port=3  Side=Right
  N_out : PMIOPort  Port=4  Side=Right
  connections:
  Capacitor/LConn1 -- Resistor1/LConn1 -- Inductor/RConn1 -- L_out/RConn1
  Inductor/LConn1 -- Resistor/RConn1
  L_in/RConn1 -- Resistor/LConn1
  Resistor1/RConn1 -- N_in/RConn1 -- N_out/RConn1 -- Capacitor/RConn1

== system Wanderwellen_Leitungsmodell/10 Leitungs-ESBs Nr. 5/Leitungs-ESB 3 ==
  Capacitor : fl_lib/Electrical/Electrical Elements/Capacitor  c=Delta_C F  r=1e-6 Ohm  g=0 1/Ohm  i_specify=off  i_priority=None  i=0 A  i_nominal_specify=off  i_nominal_unit=A  i_nominal_value=1  v_specify=off  v_priority=None  v=0 V  v_nominal_specify=off  v_nominal_unit=V  v_nominal_value=1  vc_specify=off  vc_priority=High  vc=0 V  vc_nominal_specify=off  vc_nominal_unit=V  vc_nominal_value=1
      settings: SourceProductBaseCode=PW,SS,VE
  Inductor : fl_lib/Electrical/Electrical Elements/Inductor  l=Delta_L H  r=0 Ohm  g=1e-9 1/Ohm  i_specify=off  i_priority=None  i=0 A  i_nominal_specify=off  i_nominal_unit=A  i_nominal_value=1  v_specify=off  v_priority=None  v=0 V  v_nominal_specify=off  v_nominal_unit=V  v_nominal_value=1  i_L_specify=off  i_L_priority=High  i_L=0 A  i_L_nominal_specify=off  i_L_nominal_unit=A  i_L_nominal_value=1
      settings: SourceProductBaseCode=PW,SS,VE
  Resistor : fl_lib/Electrical/Electrical Elements/Resistor  R=Delta_R Ohm  i_specify=off  i_priority=None  i=0 A  i_nominal_specify=off  i_nominal_unit=A  i_nominal_value=1  v_specify=off  v_priority=None  v=0 V  v_nominal_specify=off  v_nominal_unit=V  v_nominal_value=1
      settings: SourceProductBaseCode=PW,SS,VE
  Resistor1 : fl_lib/Electrical/Electrical Elements/Resistor  R=Delta_G Ohm  i_specify=off  i_priority=None  i=0 A  i_nominal_specify=off  i_nominal_unit=A  i_nominal_value=1  v_specify=off  v_priority=None  v=0 V  v_nominal_specify=off  v_nominal_unit=V  v_nominal_value=1
      settings: SourceProductBaseCode=PW,SS,VE
  L_in : PMIOPort  Side=Left
  N_in : PMIOPort  Port=2  Side=Left
  L_out : PMIOPort  Port=3  Side=Right
  N_out : PMIOPort  Port=4  Side=Right
  connections:
  Capacitor/LConn1 -- Resistor1/LConn1 -- Inductor/RConn1 -- L_out/RConn1
  Inductor/LConn1 -- Resistor/RConn1
  L_in/RConn1 -- Resistor/LConn1
  Resistor1/RConn1 -- N_in/RConn1 -- N_out/RConn1 -- Capacitor/RConn1

== system Wanderwellen_Leitungsmodell/10 Leitungs-ESBs Nr. 5/Leitungs-ESB 4 ==
  Capacitor : fl_lib/Electrical/Electrical Elements/Capacitor  c=Delta_C F  r=1e-6 Ohm  g=0 1/Ohm  i_specify=off  i_priority=None  i=0 A  i_nominal_specify=off  i_nominal_unit=A  i_nominal_value=1  v_specify=off  v_priority=None  v=0 V  v_nominal_specify=off  v_nominal_unit=V  v_nominal_value=1  vc_specify=off  vc_priority=High  vc=0 V  vc_nominal_specify=off  vc_nominal_unit=V  vc_nominal_value=1
      settings: SourceProductBaseCode=PW,SS,VE
  Inductor : fl_lib/Electrical/Electrical Elements/Inductor  l=Delta_L H  r=0 Ohm  g=1e-9 1/Ohm  i_specify=off  i_priority=None  i=0 A  i_nominal_specify=off  i_nominal_unit=A  i_nominal_value=1  v_specify=off  v_priority=None  v=0 V  v_nominal_specify=off  v_nominal_unit=V  v_nominal_value=1  i_L_specify=off  i_L_priority=High  i_L=0 A  i_L_nominal_specify=off  i_L_nominal_unit=A  i_L_nominal_value=1
      settings: SourceProductBaseCode=PW,SS,VE
  Resistor : fl_lib/Electrical/Electrical Elements/Resistor  R=Delta_R Ohm  i_specify=off  i_priority=None  i=0 A  i_nominal_specify=off  i_nominal_unit=A  i_nominal_value=1  v_specify=off  v_priority=None  v=0 V  v_nominal_specify=off  v_nominal_unit=V  v_nominal_value=1
      settings: SourceProductBaseCode=PW,SS,VE
  Resistor1 : fl_lib/Electrical/Electrical Elements/Resistor  R=Delta_G Ohm  i_specify=off  i_priority=None  i=0 A  i_nominal_specify=off  i_nominal_unit=A  i_nominal_value=1  v_specify=off  v_priority=None  v=0 V  v_nominal_specify=off  v_nominal_unit=V  v_nominal_value=1
      settings: SourceProductBaseCode=PW,SS,VE
  L_in : PMIOPort  Side=Left
  N_in : PMIOPort  Port=2  Side=Left
  L_out : PMIOPort  Port=3  Side=Right
  N_out : PMIOPort  Port=4  Side=Right
  connections:
  Capacitor/LConn1 -- Resistor1/LConn1 -- Inductor/RConn1 -- L_out/RConn1
  Inductor/LConn1 -- Resistor/RConn1
  L_in/RConn1 -- Resistor/LConn1
  Resistor1/RConn1 -- N_in/RConn1 -- N_out/RConn1 -- Capacitor/RConn1

== system Wanderwellen_Leitungsmodell/10 Leitungs-ESBs Nr. 5/Leitungs-ESB 5 ==
  Capacitor : fl_lib/Electrical/Electrical Elements/Capacitor  c=Delta_C F  r=1e-6 Ohm  g=0 1/Ohm  i_specify=off  i_priority=None  i=0 A  i_nominal_specify=off  i_nominal_unit=A  i_nominal_value=1  v_specify=off  v_priority=None  v=0 V  v_nominal_specify=off  v_nominal_unit=V  v_nominal_value=1  vc_specify=off  vc_priority=High  vc=0 V  vc_nominal_specify=off  vc_nominal_unit=V  vc_nominal_value=1
      settings: SourceProductBaseCode=PW,SS,VE
  Inductor : fl_lib/Electrical/Electrical Elements/Inductor  l=Delta_L H  r=0 Ohm  g=1e-9 1/Ohm  i_specify=off  i_priority=None  i=0 A  i_nominal_specify=off  i_nominal_unit=A  i_nominal_value=1  v_specify=off  v_priority=None  v=0 V  v_nominal_specify=off  v_nominal_unit=V  v_nominal_value=1  i_L_specify=off  i_L_priority=High  i_L=0 A  i_L_nominal_specify=off  i_L_nominal_unit=A  i_L_nominal_value=1
      settings: SourceProductBaseCode=PW,SS,VE
  Resistor : fl_lib/Electrical/Electrical Elements/Resistor  R=Delta_R Ohm  i_specify=off  i_priority=None  i=0 A  i_nominal_specify=off  i_nominal_unit=A  i_nominal_value=1  v_specify=off  v_priority=None  v=0 V  v_nominal_specify=off  v_nominal_unit=V  v_nominal_value=1
      settings: SourceProductBaseCode=PW,SS,VE
  Resistor1 : fl_lib/Electrical/Electrical Elements/Resistor  R=Delta_G Ohm  i_specify=off  i_priority=None  i=0 A  i_nominal_specify=off  i_nominal_unit=A  i_nominal_value=1  v_specify=off  v_priority=None  v=0 V  v_nominal_specify=off  v_nominal_unit=V  v_nominal_value=1
      settings: SourceProductBaseCode=PW,SS,VE
  L_in : PMIOPort  Side=Left
  N_in : PMIOPort  Port=2  Side=Left
  L_out : PMIOPort  Port=3  Side=Right
  N_out : PMIOPort  Port=4  Side=Right
  connections:
  Capacitor/LConn1 -- Resistor1/LConn1 -- Inductor/RConn1 -- L_out/RConn1
  Inductor/LConn1 -- Resistor/RConn1
  L_in/RConn1 -- Resistor/LConn1
  Resistor1/RConn1 -- N_in/RConn1 -- N_out/RConn1 -- Capacitor/RConn1

== system Wanderwellen_Leitungsmodell/10 Leitungs-ESBs Nr. 5/Leitungs-ESB 6 ==
  Capacitor : fl_lib/Electrical/Electrical Elements/Capacitor  c=Delta_C F  r=1e-6 Ohm  g=0 1/Ohm  i_specify=off  i_priority=None  i=0 A  i_nominal_specify=off  i_nominal_unit=A  i_nominal_value=1  v_specify=off  v_priority=None  v=0 V  v_nominal_specify=off  v_nominal_unit=V  v_nominal_value=1  vc_specify=off  vc_priority=High  vc=0 V  vc_nominal_specify=off  vc_nominal_unit=V  vc_nominal_value=1
      settings: SourceProductBaseCode=PW,SS,VE
  Inductor : fl_lib/Electrical/Electrical Elements/Inductor  l=Delta_L H  r=0 Ohm  g=1e-9 1/Ohm  i_specify=off  i_priority=None  i=0 A  i_nominal_specify=off  i_nominal_unit=A  i_nominal_value=1  v_specify=off  v_priority=None  v=0 V  v_nominal_specify=off  v_nominal_unit=V  v_nominal_value=1  i_L_specify=off  i_L_priority=High  i_L=0 A  i_L_nominal_specify=off  i_L_nominal_unit=A  i_L_nominal_value=1
      settings: SourceProductBaseCode=PW,SS,VE
  Resistor : fl_lib/Electrical/Electrical Elements/Resistor  R=Delta_R Ohm  i_specify=off  i_priority=None  i=0 A  i_nominal_specify=off  i_nominal_unit=A  i_nominal_value=1  v_specify=off  v_priority=None  v=0 V  v_nominal_specify=off  v_nominal_unit=V  v_nominal_value=1
      settings: SourceProductBaseCode=PW,SS,VE
  Resistor1 : fl_lib/Electrical/Electrical Elements/Resistor  R=Delta_G Ohm  i_specify=off  i_priority=None  i=0 A  i_nominal_specify=off  i_nominal_unit=A  i_nominal_value=1  v_specify=off  v_priority=None  v=0 V  v_nominal_specify=off  v_nominal_unit=V  v_nominal_value=1
      settings: SourceProductBaseCode=PW,SS,VE
  L_in : PMIOPort  Side=Left
  N_in : PMIOPort  Port=2  Side=Left
  L_out : PMIOPort  Port=3  Side=Right
  N_out : PMIOPort  Port=4  Side=Right
  connections:
  Capacitor/LConn1 -- Resistor1/LConn1 -- Inductor/RConn1 -- L_out/RConn1
  Inductor/LConn1 -- Resistor/RConn1
  L_in/RConn1 -- Resistor/LConn1
  Resistor1/RConn1 -- N_in/RConn1 -- N_out/RConn1 -- Capacitor/RConn1

== system Wanderwellen_Leitungsmodell/10 Leitungs-ESBs Nr. 5/Leitungs-ESB 7 ==
  Capacitor : fl_lib/Electrical/Electrical Elements/Capacitor  c=Delta_C F  r=1e-6 Ohm  g=0 1/Ohm  i_specify=off  i_priority=None  i=0 A  i_nominal_specify=off  i_nominal_unit=A  i_nominal_value=1  v_specify=off  v_priority=None  v=0 V  v_nominal_specify=off  v_nominal_unit=V  v_nominal_value=1  vc_specify=off  vc_priority=High  vc=0 V  vc_nominal_specify=off  vc_nominal_unit=V  vc_nominal_value=1
      settings: SourceProductBaseCode=PW,SS,VE
  Inductor : fl_lib/Electrical/Electrical Elements/Inductor  l=Delta_L H  r=0 Ohm  g=1e-9 1/Ohm  i_specify=off  i_priority=None  i=0 A  i_nominal_specify=off  i_nominal_unit=A  i_nominal_value=1  v_specify=off  v_priority=None  v=0 V  v_nominal_specify=off  v_nominal_unit=V  v_nominal_value=1  i_L_specify=off  i_L_priority=High  i_L=0 A  i_L_nominal_specify=off  i_L_nominal_unit=A  i_L_nominal_value=1
      settings: SourceProductBaseCode=PW,SS,VE
  Resistor : fl_lib/Electrical/Electrical Elements/Resistor  R=Delta_R Ohm  i_specify=off  i_priority=None  i=0 A  i_nominal_specify=off  i_nominal_unit=A  i_nominal_value=1  v_specify=off  v_priority=None  v=0 V  v_nominal_specify=off  v_nominal_unit=V  v_nominal_value=1
      settings: SourceProductBaseCode=PW,SS,VE
  Resistor1 : fl_lib/Electrical/Electrical Elements/Resistor  R=Delta_G Ohm  i_specify=off  i_priority=None  i=0 A  i_nominal_specify=off  i_nominal_unit=A  i_nominal_value=1  v_specify=off  v_priority=None  v=0 V  v_nominal_specify=off  v_nominal_unit=V  v_nominal_value=1
      settings: SourceProductBaseCode=PW,SS,VE
  L_in : PMIOPort  Side=Left
  N_in : PMIOPort  Port=2  Side=Left
  L_out : PMIOPort  Port=3  Side=Right
  N_out : PMIOPort  Port=4  Side=Right
  connections:
  Capacitor/LConn1 -- Resistor1/LConn1 -- Inductor/RConn1 -- L_out/RConn1
  Inductor/LConn1 -- Resistor/RConn1
  L_in/RConn1 -- Resistor/LConn1
  Resistor1/RConn1 -- N_in/RConn1 -- N_out/RConn1 -- Capacitor/RConn1

== system Wanderwellen_Leitungsmodell/10 Leitungs-ESBs Nr. 5/Leitungs-ESB 8 ==
  Capacitor : fl_lib/Electrical/Electrical Elements/Capacitor  c=Delta_C F  r=1e-6 Ohm  g=0 1/Ohm  i_specify=off  i_priority=None  i=0 A  i_nominal_specify=off  i_nominal_unit=A  i_nominal_value=1  v_specify=off  v_priority=None  v=0 V  v_nominal_specify=off  v_nominal_unit=V  v_nominal_value=1  vc_specify=off  vc_priority=High  vc=0 V  vc_nominal_specify=off  vc_nominal_unit=V  vc_nominal_value=1
      settings: SourceProductBaseCode=PW,SS,VE
  Inductor : fl_lib/Electrical/Electrical Elements/Inductor  l=Delta_L H  r=0 Ohm  g=1e-9 1/Ohm  i_specify=off  i_priority=None  i=0 A  i_nominal_specify=off  i_nominal_unit=A  i_nominal_value=1  v_specify=off  v_priority=None  v=0 V  v_nominal_specify=off  v_nominal_unit=V  v_nominal_value=1  i_L_specify=off  i_L_priority=High  i_L=0 A  i_L_nominal_specify=off  i_L_nominal_unit=A  i_L_nominal_value=1
      settings: SourceProductBaseCode=PW,SS,VE
  Resistor : fl_lib/Electrical/Electrical Elements/Resistor  R=Delta_R Ohm  i_specify=off  i_priority=None  i=0 A  i_nominal_specify=off  i_nominal_unit=A  i_nominal_value=1  v_specify=off  v_priority=None  v=0 V  v_nominal_specify=off  v_nominal_unit=V  v_nominal_value=1
      settings: SourceProductBaseCode=PW,SS,VE
  Resistor1 : fl_lib/Electrical/Electrical Elements/Resistor  R=Delta_G Ohm  i_specify=off  i_priority=None  i=0 A  i_nominal_specify=off  i_nominal_unit=A  i_nominal_value=1  v_specify=off  v_priority=None  v=0 V  v_nominal_specify=off  v_nominal_unit=V  v_nominal_value=1
      settings: SourceProductBaseCode=PW,SS,VE
  L_in : PMIOPort  Side=Left
  N_in : PMIOPort  Port=2  Side=Left
  L_out : PMIOPort  Port=3  Side=Right
  N_out : PMIOPort  Port=4  Side=Right
  connections:
  Capacitor/LConn1 -- Resistor1/LConn1 -- Inductor/RConn1 -- L_out/RConn1
  Inductor/LConn1 -- Resistor/RConn1
  L_in/RConn1 -- Resistor/LConn1
  Resistor1/RConn1 -- N_in/RConn1 -- N_out/RConn1 -- Capacitor/RConn1

== system Wanderwellen_Leitungsmodell/10 Leitungs-ESBs Nr. 5/Leitungs-ESB 9 ==
  Capacitor : fl_lib/Electrical/Electrical Elements/Capacitor  c=Delta_C F  r=1e-6 Ohm  g=0 1/Ohm  i_specify=off  i_priority=None  i=0 A  i_nominal_specify=off  i_nominal_unit=A  i_nominal_value=1  v_specify=off  v_priority=None  v=0 V  v_nominal_specify=off  v_nominal_unit=V  v_nominal_value=1  vc_specify=off  vc_priority=High  vc=0 V  vc_nominal_specify=off  vc_nominal_unit=V  vc_nominal_value=1
      settings: SourceProductBaseCode=PW,SS,VE
  Inductor : fl_lib/Electrical/Electrical Elements/Inductor  l=Delta_L H  r=0 Ohm  g=1e-9 1/Ohm  i_specify=off  i_priority=None  i=0 A  i_nominal_specify=off  i_nominal_unit=A  i_nominal_value=1  v_specify=off  v_priority=None  v=0 V  v_nominal_specify=off  v_nominal_unit=V  v_nominal_value=1  i_L_specify=off  i_L_priority=High  i_L=0 A  i_L_nominal_specify=off  i_L_nominal_unit=A  i_L_nominal_value=1
      settings: SourceProductBaseCode=PW,SS,VE
  Resistor : fl_lib/Electrical/Electrical Elements/Resistor  R=Delta_R Ohm  i_specify=off  i_priority=None  i=0 A  i_nominal_specify=off  i_nominal_unit=A  i_nominal_value=1  v_specify=off  v_priority=None  v=0 V  v_nominal_specify=off  v_nominal_unit=V  v_nominal_value=1
      settings: SourceProductBaseCode=PW,SS,VE
  Resistor1 : fl_lib/Electrical/Electrical Elements/Resistor  R=Delta_G Ohm  i_specify=off  i_priority=None  i=0 A  i_nominal_specify=off  i_nominal_unit=A  i_nominal_value=1  v_specify=off  v_priority=None  v=0 V  v_nominal_specify=off  v_nominal_unit=V  v_nominal_value=1
      settings: SourceProductBaseCode=PW,SS,VE
  L_in : PMIOPort  Side=Left
  N_in : PMIOPort  Port=2  Side=Left
  L_out : PMIOPort  Port=3  Side=Right
  N_out : PMIOPort  Port=4  Side=Right
  connections:
  Capacitor/LConn1 -- Resistor1/LConn1 -- Inductor/RConn1 -- L_out/RConn1
  Inductor/LConn1 -- Resistor/RConn1
  L_in/RConn1 -- Resistor/LConn1
  Resistor1/RConn1 -- N_in/RConn1 -- N_out/RConn1 -- Capacitor/RConn1
